simulink model "E5"  (R2023a)
settings: Solver=VariableStepAuto  StartTime=0.0  StopTime=0.08  MaxStep=1e-4  RelTol=1e-3
libraries: spsDetailedThyristorLib x6, spsACVoltageSourceLib x3, spsGroundLib x1, spsMeanLib x1, spsSeriesRLCBranchLib x1, spsVoltageMeasurementLib x1, sps_lib x1
settings Model: Creator=swara  LastModifiedBy=swara

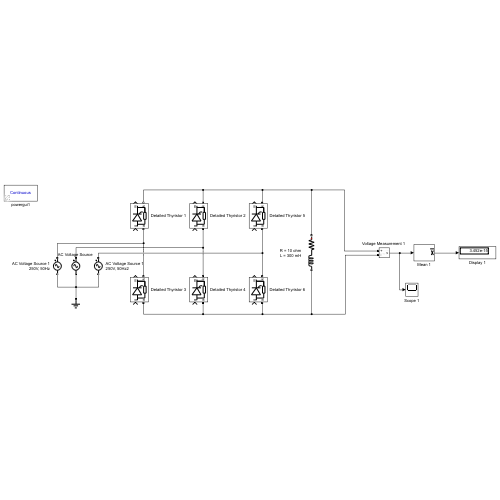
[thumbnail: Simulink's stored preview of the top-level diagram]
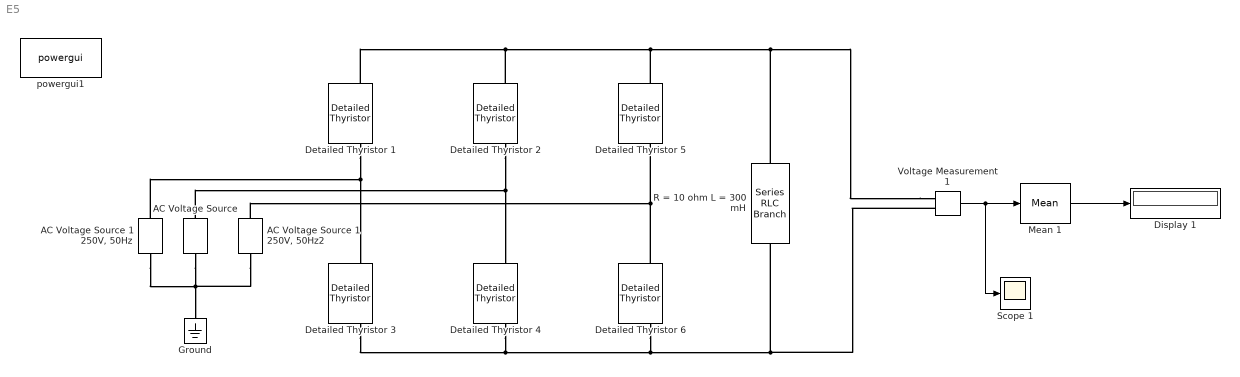
== system E5 ==
  "AC Voltage Source " : spsACVoltageSourceLib/AC Voltage Source  Amplitude=250  Phase=120  Frequency=50  SampleTime=0  Measurements=None  BusType=swing  Pref=10e3  Qref=0  Qmin=-inf  Qmax=+inf
  "AC Voltage Source 1 250V, 50Hz" : spsACVoltageSourceLib/AC Voltage Source  Amplitude=250  Phase=0  Frequency=50  SampleTime=0  Measurements=None  BusType=swing  Pref=10e3  Qref=0  Qmin=-inf  Qmax=+inf
  "AC Voltage Source 1 250V, 50Hz2" : spsACVoltageSourceLib/AC Voltage Source  Amplitude=250  Phase=240  Frequency=50  SampleTime=0  Measurements=None  BusType=swing  Pref=10e3  Qref=0  Qmin=-inf  Qmax=+inf
  Detailed Thyristor {1..6} (6 alike) : spsDetailedThyristorLib/Detailed Thyristor  Ron=0.001  Lon=1e-3  Vf=0.8  IL=0.1  Tq=100e-6  IC=0  Rs=500  Cs=250e-9  Measurements=on
      settings: LibrarySourceBlock=sps_lib/Power Electronics/Detailed Thyristor
  Display 1 : Display
  Ground : spsGroundLib/Ground  LConnTagsString=a
  Mean 1 : spsMeanLib/Mean  Freq=50  Vinit=0  Ts=0
  R = 10 ohm L = 300 mH : spsSeriesRLCBranchLib/Series RLC Branch  LConnTagsString=__new0  RConnTagsString=__new0  BranchType=RL  Resistance=10  Inductance=3  SetiL0=off  InitialCurrent=0  Capacitance=1e-6  Setx0=off  InitialVoltage=0  Measurements=None
  Scope 1 : Scope
  "Voltage Measurement 1 " : spsVoltageMeasurementLib/Voltage Measurement  PhasorSimulation=off  OutputType=Complex  PSBequivalent=0
  powergui1 : sps_lib/powergui  Priority=1  SimulationMode=Continuous  SampleTime=50e-6  frequency=60  Iterations=50  frequencyindice=50  Pbase=100e6  ErrMax=1e-4  UnitsV=kV  UnitsW=MW  buscounter=0  FunctionMessages=off  echomessages=off  EnableUseOfTLC=off  CurrentSourceSwitches=off  DisableSnubberDevices=off  DisableRonSwitches=off  DisableVfSwitches=off  DisplayEquations=off  AutomaticDiscreteSolvers=off  SolverType=Tustin/Backward Euler (TBE)  Interpol=off  ExternalGateDelay=off  methode=off  Ts=100  x0status=zero  SPID=on  SwTol=0  HookPort=off  NonlinearTolerance=1e-4  nMaxIteration=100  ContinueOnMaxIteration=off  RestoreLinks=warning  ResistiveCurrentMeasurement=off  Frange=[0:2:500]  Ylog=off  Xlog=on  ShowGrid=off  save=off  variable=ZData  structure=0  ZoomFFT=off  StartTime=0.0  cycles=1  DisplayStyle=1  fundamental=60  FreqAxis=off  MaxFrequency=1000  frequencyindicesteady=1  RmsSteady=1  display=off
  wires:
  "Voltage Measurement 1 "/1 -> Scope 1/1, Mean 1/1
  Mean 1/1 -> Display 1/1
  connections:
  R = 10 ohm L = 300 mH/RConn1 -- Detailed Thyristor 3/LConn1 -- Detailed Thyristor 4/LConn1 -- Detailed Thyristor 6/LConn1 -- "Voltage Measurement 1 "/LConn2
  "AC Voltage Source 1 250V, 50Hz"/RConn1 -- Detailed Thyristor 1/LConn1 -- Detailed Thyristor 3/RConn1
  Detailed Thyristor 2/LConn1 -- "AC Voltage Source "/RConn1 -- Detailed Thyristor 4/RConn1
  "Voltage Measurement 1 "/LConn1 -- Detailed Thyristor 5/RConn1 -- Detailed Thyristor 2/RConn1 -- Detailed Thyristor 1/RConn1 -- R = 10 ohm L = 300 mH/LConn1
  Detailed Thyristor 6/RConn1 -- Detailed Thyristor 5/LConn1 -- "AC Voltage Source 1 250V, 50Hz2"/RConn1
  "AC Voltage Source "/LConn1 -- "AC Voltage Source 1 250V, 50Hz"/LConn1 -- Ground/LConn1 -- "AC Voltage Source 1 250V, 50Hz2"/LConn1
